simulink model "p_pd_regler_alleine"  (R2016b)
settings: Solver=FixedStepAuto  StartTime=0.0  StopTime=50.0  FixedStep=0.01  RelTol=1e-3
values from neighbouring files (symbols this model uses):
  T_N = 1    [real_pd.m]
  T_R = 2    [real_pd.m]
undefined symbols (not defined in the file or in its folder): K_D, K_P, transfunc
settings Model: Creator=Fritz  LastModifiedBy=Fritz

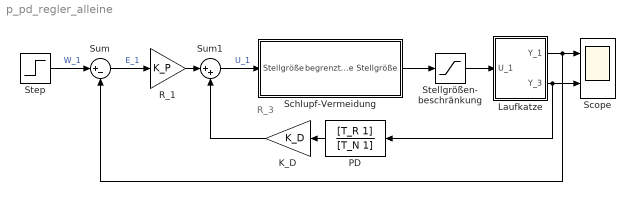
== system p_pd_regler_alleine ==
  note: R_3
  K_D : Gain  Gain=K_D
  Laufkatze : Subsystem
  PD : TransferFcn  Numerator=[T_R 1]  Denominator=[T_N 1]
  R_1 : Gain  Gain=K_P
  Schlupf-Vermeidung : Subsystem
  Scope : Scope  NumInputPorts=2
  Stellgrößen- beschränkung : Saturate  UpperLimit=75  LowerLimit=-75
  Step : Step  Time=0  SampleTime=0
  Sum : Sum  Inputs=|+-
  Sum1 : Sum  Inputs=|++
  wires:
  Step/1 -> Sum/1  "W_1"
  Schlupf-Vermeidung/1(begrenzte Stellgröße) -> Stellgrößen- beschränkung/1
  Sum/1 -> R_1/1  "E_1"
  Laufkatze/1(Y_1) -> Sum/2, Scope/1
  Stellgrößen- beschränkung/1 -> Laufkatze/1(U_1)
  R_1/1 -> Sum1/1
  Sum1/1 -> Schlupf-Vermeidung/1(Stellgröße)  "U_1"
  K_D/1 -> Sum1/2
  Laufkatze/2(Y_3) -> PD/1, Scope/2
  PD/1 -> K_D/1

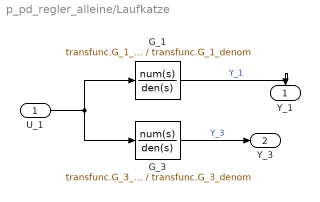
== system p_pd_regler_alleine/Laufkatze ==
  U_1 : Inport
  G_1 : TransferFcn  Numerator=transfunc.G_1_numer  Denominator=transfunc.G_1_denom
  G_3 : TransferFcn  Numerator=transfunc.G_3_numer  Denominator=transfunc.G_3_denom
  Y_1 : Outport
  Y_3 : Outport  Port=2
  wires:
  U_1/1 -> G_3/1, G_1/1
  G_3/1 -> Y_3/1  "Y_3"
  G_1/1 -> Y_1/1  "Y_1"

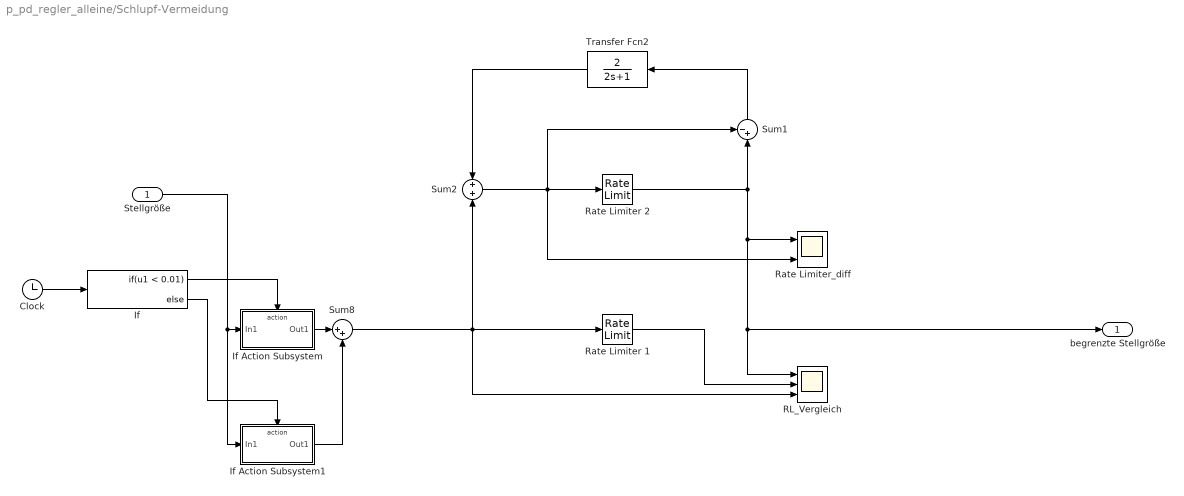
== system p_pd_regler_alleine/Schlupf-Vermeidung ==
  Stellgröße : Inport
  Clock : Clock
  If : If  IfExpression=u1 < 0.01
  If Action Subsystem : Subsystem  TreatAsAtomicUnit=on
  If Action Subsystem1 : Subsystem  TreatAsAtomicUnit=on
  RL_Vergleich : Scope  NumInputPorts=3
  Rate Limiter 1 : RateLimiter  RisingSlewLimit=9.57  FallingSlewLimit=-9.57  SampleTimeMode=inherited
  Rate Limiter 2 : RateLimiter  RisingSlewLimit=9.57  FallingSlewLimit=-9.57  SampleTimeMode=inherited
  Rate Limiter_diff : Scope  NumInputPorts=2
  Sum1 : Sum  Inputs=-+|
  Sum2 : Sum  Inputs=+|+
  Sum8 : Sum  Inputs=|++
  Transfer Fcn2 : TransferFcn  Numerator=[2]  Denominator=[2 1]
  begrenzte Stellgröße : Outport
  wires:
  Stellgröße/1 -> If Action Subsystem1/1(In1), If Action Subsystem/1(In1)
  If Action Subsystem/1(Out1) -> Sum8/1
  If Action Subsystem1/1(Out1) -> Sum8/2
  Clock/1 -> If/1
  If/1 -> If Action Subsystem/Action
  If/2 -> If Action Subsystem1/Action
  Sum8/1 -> RL_Vergleich/3, Sum2/2, Rate Limiter 1/1
  Sum2/1 -> Rate Limiter_diff/2, Sum1/1, Rate Limiter 2/1
  Sum1/1 -> Transfer Fcn2/1
  Transfer Fcn2/1 -> Sum2/1
  Rate Limiter 2/1 -> begrenzte Stellgröße/1, RL_Vergleich/1, Rate Limiter_diff/1, Sum1/2
  Rate Limiter 1/1 -> RL_Vergleich/2

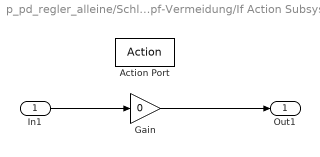
== system p_pd_regler_alleine/Schlupf-Vermeidung/If Action Subsystem ==
  In1 : Inport
  Action Port : ActionPort  ActionType=then
  Gain : Gain  Gain=0
  Out1 : Outport
  wires:
  In1/1 -> Gain/1
  Gain/1 -> Out1/1

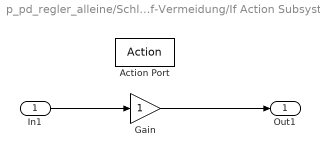
== system p_pd_regler_alleine/Schlupf-Vermeidung/If Action Subsystem1 ==
  In1 : Inport
  Action Port : ActionPort  ActionType=else
  Gain : Gain
  Out1 : Outport
  wires:
  In1/1 -> Gain/1
  Gain/1 -> Out1/1
